simulink model "multi_module_phase_shift_generator_base"  (R2025b)
settings: Solver=FixedStepDiscrete  StartTime=0.0  StopTime=10e3  RelTol=1e-3
libraries: simulink x3
settings Model: DataTypeOverride=Off  Creator=KoayXianCong  LastModifiedBy=KoayXianCong
settings OptimizationCC: BlockReduction=off  ConditionallyExecuteInputs=off  DefaultParameterBehavior=Inlined  InheritOutputTypeSmallerThanSingle=on
settings DebuggingCC: SignalRangeChecking=warning  ArtificialAlgebraicLoopMsg=error  SingleTaskRateTransMsg=error
settings HardwareCC: ProdBitPerPointer=32.0  ProdBitPerSizeT=32.0  ProdBitPerPtrDiffT=32.0  ProdLargestAtomicFloat=None  ProdIntDivRoundTo=Undefined  ProdEndianess=Unspecified  ProdWordSize=32.0  ProdHWDeviceType=ASIC/FPGA->ASIC/FPGA  TargetBitPerPointer=64.0  TargetBitPerSizeT=64.0  TargetBitPerPtrDiffT=64.0  TargetLongLongMode=on  TargetIntDivRoundTo=Zero  TargetEndianess=LittleEndian  TargetWordSize=64.0  TargetHWDeviceType=Custom Processor->MATLAB Host Computer  ProdEqTarget=off

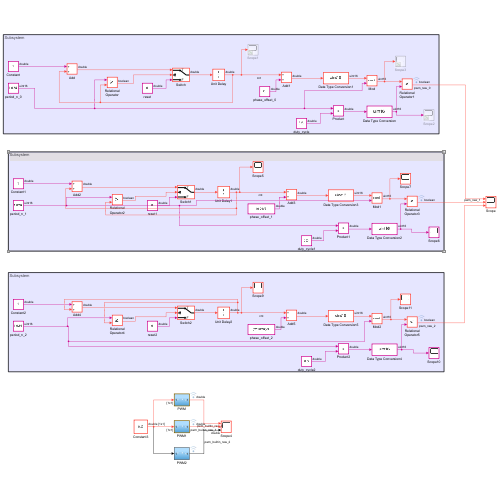
[thumbnail: Simulink's stored preview of the top-level diagram]
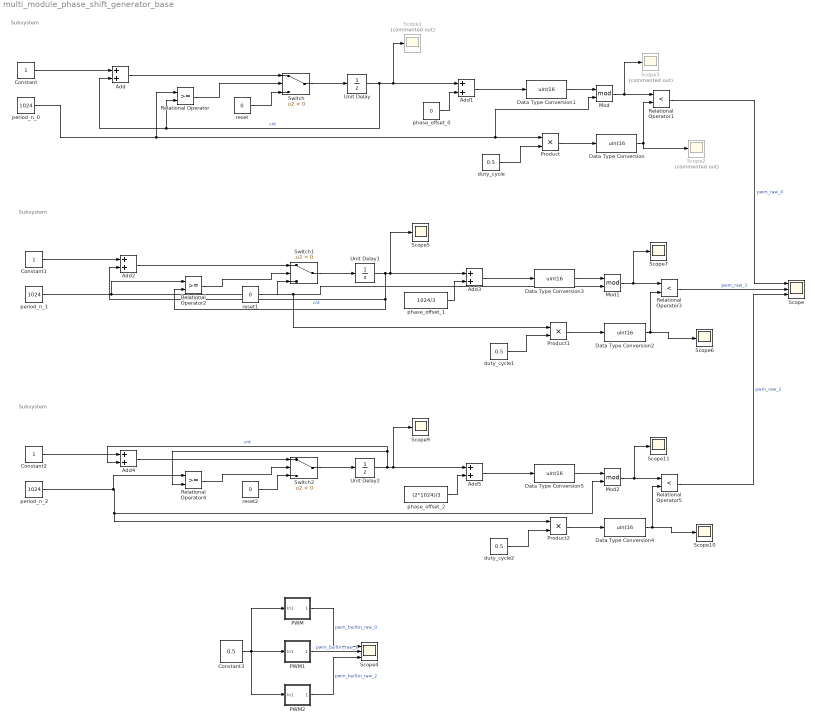
== system multi_module_phase_shift_generator_base ==
  note: Subsystem
  note: Subsystem
  note: Subsystem
  Add{,1..5} (6 alike) : Sum
  Constant : Constant
  Constant1 : Constant
  Constant2 : Constant
  Constant3 : Constant  Value=0.5  VectorParams1D=off  SampleTime=1
  Data Type Conversion{,1..5} (6 alike) : DataTypeConversion  OutDataTypeStr=uint16  SaturateOnIntegerOverflow=off  RndMeth=Floor
  Mod : Math  Operator=mod
  Mod1 : Math  Operator=mod
  Mod2 : Math  Operator=mod
  PWM : Subsystem  Tag=DecoupledSystem
  PWM1 : Subsystem  Tag=DecoupledSystem
  PWM2 : Subsystem  Tag=DecoupledSystem
  Product : Product
  Product1 : Product
  Product2 : Product
  Relational Operator : RelationalOperator  OutDataTypeStr=boolean  RndMeth=Simplest  InputSameDT=off
  Relational Operator1 : RelationalOperator  Operator=<  OutDataTypeStr=boolean  RndMeth=Simplest  InputSameDT=off
  Relational Operator2 : RelationalOperator  OutDataTypeStr=boolean  RndMeth=Simplest  InputSameDT=off
  Relational Operator3 : RelationalOperator  Operator=<  OutDataTypeStr=boolean  RndMeth=Simplest  InputSameDT=off
  Relational Operator4 : RelationalOperator  OutDataTypeStr=boolean  RndMeth=Simplest  InputSameDT=off
  Relational Operator5 : RelationalOperator  Operator=<  OutDataTypeStr=boolean  RndMeth=Simplest  InputSameDT=off
  Scope : Scope  NumInputPorts=3
      settings: ActiveDisplayYMinimum=0.34102183262647323  ActiveDisplayYMaximum=0.598106128125198
  Scope1 : Scope  Commented=on
      settings: ActiveDisplayYMinimum=-128.12499999999997  ActiveDisplayYMaximum=1153.125
  Scope{5..7,9..11} (6 alike) : Scope
      Scope10 settings: ActiveDisplayYMinimum=506.79812224932584  ActiveDisplayYMaximum=514.31790981439906  DataLoggingVariableName=ScopeData8
      Scope11 settings: ActiveDisplayYMinimum=-7.9410266457680265  ActiveDisplayYMaximum=60.965223354231973  DataLoggingVariableName=ScopeData9
      Scope5 settings: ActiveDisplayYMinimum=-128.12499999999997  ActiveDisplayYMaximum=1153.125  DataLoggingVariableName=ScopeData5
      Scope6 settings: ActiveDisplayYMinimum=506.79812224932584  ActiveDisplayYMaximum=514.31790981439906  DataLoggingVariableName=ScopeData6
      Scope7 settings: ActiveDisplayYMinimum=-7.9410266457680265  ActiveDisplayYMaximum=60.965223354231973  DataLoggingVariableName=ScopeData7
      Scope9 settings: ActiveDisplayYMinimum=-128.12499999999997  ActiveDisplayYMaximum=1153.125  DataLoggingVariableName=ScopeData11
  Scope2 : Scope  Commented=on
      settings: ActiveDisplayYMinimum=506.79812224932584  ActiveDisplayYMaximum=514.31790981439906  DataLoggingVariableName=ScopeData2
  Scope3 : Scope  Commented=on
      settings: ActiveDisplayYMinimum=-7.9410266457680265  ActiveDisplayYMaximum=60.965223354231973  DataLoggingVariableName=ScopeData3
  Scope4 : Scope  NumInputPorts=3
      settings: ActiveDisplayYMinimum=-0.15719261881639313  ActiveDisplayYMaximum=1.3621901936836069  DataLoggingVariableName=ScopeData4  DataLoggingSaveFormat=Array
  Switch : Switch  Criteria=u2 > Threshold  SaturateOnIntegerOverflow=off  InputSameDT=off
  Switch1 : Switch  Criteria=u2 > Threshold  SaturateOnIntegerOverflow=off  InputSameDT=off
  Switch2 : Switch  Criteria=u2 > Threshold  SaturateOnIntegerOverflow=off  InputSameDT=off
  Unit Delay : UnitDelay  HasFrameUpgradeWarning=on
  Unit Delay1 : UnitDelay  HasFrameUpgradeWarning=on
  Unit Delay2 : UnitDelay  HasFrameUpgradeWarning=on
  duty_cycle : Constant  Value=0.5
  duty_cycle1 : Constant  Value=0.5
  duty_cycle2 : Constant  Value=0.5
  period_n_0 : Constant  Value=1024  OutDataTypeStr=uint16
  period_n_1 : Constant  Value=1024  OutDataTypeStr=uint16
  period_n_2 : Constant  Value=1024  OutDataTypeStr=uint16
  phase_offset_0 : Constant  Value=0
  phase_offset_1 : Constant  Value=1024/3
  phase_offset_2 : Constant  Value=(2*1024)/3
  reset : Constant  Value=0
  reset1 : Constant  Value=0
  reset2 : Constant  Value=0
  wires:
  Add1/1 -> Data Type Conversion1/1
  Relational Operator1/1 -> Scope/1  "pwm_raw_0"
  Constant/1 -> Add/1
  Add/1 -> Switch/1
  duty_cycle/1 -> Product/2
  Switch/1 -> Unit Delay/1
  Unit Delay/1 -> Scope1/1, Add1/1, Relational Operator/2, Add/2  "cnt"
  Product/1 -> Data Type Conversion/1
  reset/1 -> Switch/3
  period_n_0/1 -> Relational Operator/1, Mod/2, Product/1
  phase_offset_0/1 -> Add1/2
  Data Type Conversion/1 -> Relational Operator1/2, Scope2/1
  Mod/1 -> Scope3/1, Relational Operator1/1
  Relational Operator/1 -> Switch/2
  Data Type Conversion1/1 -> Mod/1
  Relational Operator3/1 -> Scope/2  "pwm_raw_1"
  Product1/1 -> Data Type Conversion2/1
  Mod1/1 -> Scope7/1, Relational Operator3/1
  Add3/1 -> Data Type Conversion3/1
  Data Type Conversion3/1 -> Mod1/1
  duty_cycle1/1 -> Product1/2
  Relational Operator2/1 -> Switch1/2
  Constant1/1 -> Add2/1
  period_n_1/1 -> Mod1/2, Product1/1, Relational Operator2/1
  Add2/1 -> Switch1/1
  Unit Delay1/1 -> Relational Operator2/2, Add2/2, Scope5/1, Add3/1  "cnt"
  reset1/1 -> Switch1/3
  Switch1/1 -> Unit Delay1/1
  phase_offset_1/1 -> Add3/2
  Data Type Conversion2/1 -> Relational Operator3/2, Scope6/1
  Relational Operator5/1 -> Scope/3  "pwm_raw_2"
  duty_cycle2/1 -> Product2/2
  Data Type Conversion5/1 -> Mod2/1
  period_n_2/1 -> Mod2/2, Product2/1, Relational Operator4/1
  Add5/1 -> Data Type Conversion5/1
  Constant2/1 -> Add4/1
  Unit Delay2/1 -> Scope9/1, Add5/1, Relational Operator4/2, Add4/2  "cnt"
  Data Type Conversion4/1 -> Relational Operator5/2, Scope10/1
  Product2/1 -> Data Type Conversion4/1
  Switch2/1 -> Unit Delay2/1
  reset2/1 -> Switch2/3
  Mod2/1 -> Scope11/1, Relational Operator5/1
  Relational Operator4/1 -> Switch2/2
  phase_offset_2/1 -> Add5/2
  Add4/1 -> Switch2/1
  Constant3/1 -> PWM2/1(In1), PWM/1(In1), PWM1/1(In1)
  PWM/1(Out1) -> Scope4/1  "pwm_builtin_raw_0"
  PWM1/1(Out1) -> Scope4/2  "pwm_builtin_raw_1"
  PWM2/1(Out1) -> Scope4/3  "pwm_builtin_raw_2"

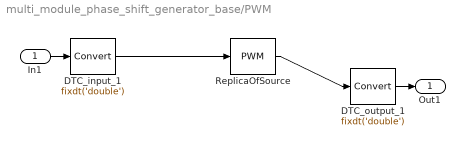
== system multi_module_phase_shift_generator_base/PWM ==
  In1 : Inport  LockScale=on
  DTC_input_1 : DataTypeConversion  OutDataTypeStr=fixdt('double')  RndMeth=Nearest  SaturateOnIntegerOverflow=off  LockScale=on
  DTC_output_1 : DataTypeConversion  OutDataTypeStr=fixdt('double')  SaturateOnIntegerOverflow=off  RndMeth=Floor
  ReplicaOfSource : simulink/Discontinuities/PWM  DisableCoverage=on  Period=1024  InitialDelay=0  DisallowZeroDutyCycle=off  RunAtFixedTimeIntervals=on  SampleTime=1
      settings: LibrarySourceBlock=hdlsllib/RCP and HIL/PWM
  Out1 : Outport  LockScale=on
  wires:
  In1/1 -> DTC_input_1/1
  DTC_output_1/1 -> Out1/1
  DTC_input_1/1 -> ReplicaOfSource/1
  ReplicaOfSource/1 -> DTC_output_1/1

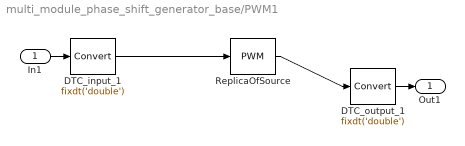
== system multi_module_phase_shift_generator_base/PWM1 ==
  In1 : Inport  LockScale=on
  DTC_input_1 : DataTypeConversion  OutDataTypeStr=fixdt('double')  RndMeth=Nearest  SaturateOnIntegerOverflow=off  LockScale=on
  DTC_output_1 : DataTypeConversion  OutDataTypeStr=fixdt('double')  SaturateOnIntegerOverflow=off  RndMeth=Floor
  ReplicaOfSource : simulink/Discontinuities/PWM  DisableCoverage=on  Period=1024  InitialDelay=1024/3  DisallowZeroDutyCycle=off  RunAtFixedTimeIntervals=on  SampleTime=1
      settings: LibrarySourceBlock=hdlsllib/RCP and HIL/PWM
  Out1 : Outport  LockScale=on
  wires:
  ReplicaOfSource/1 -> DTC_output_1/1
  DTC_output_1/1 -> Out1/1
  In1/1 -> DTC_input_1/1
  DTC_input_1/1 -> ReplicaOfSource/1

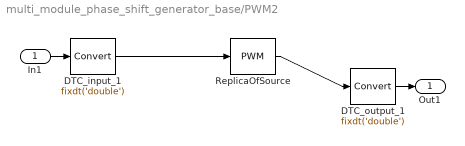
== system multi_module_phase_shift_generator_base/PWM2 ==
  In1 : Inport  LockScale=on
  DTC_input_1 : DataTypeConversion  OutDataTypeStr=fixdt('double')  RndMeth=Nearest  SaturateOnIntegerOverflow=off  LockScale=on
  DTC_output_1 : DataTypeConversion  OutDataTypeStr=fixdt('double')  SaturateOnIntegerOverflow=off  RndMeth=Floor
  ReplicaOfSource : simulink/Discontinuities/PWM  DisableCoverage=on  Period=1024  InitialDelay=(2*1024)/3  DisallowZeroDutyCycle=off  RunAtFixedTimeIntervals=on  SampleTime=1
      settings: LibrarySourceBlock=hdlsllib/RCP and HIL/PWM
  Out1 : Outport  LockScale=on
  wires:
  DTC_output_1/1 -> Out1/1
  In1/1 -> DTC_input_1/1
  DTC_input_1/1 -> ReplicaOfSource/1
  ReplicaOfSource/1 -> DTC_output_1/1
